simulink model "source"  (R2024b)
settings: Solver=ode15s  StartTime=0.0  StopTime=20  MaxStep=base.Ts  RelTol=1e-3  AbsTol=1e-4
values from neighbouring files (symbols this model uses):
  base = evalin("base", "base")    [base_wheel_state_space.m]    (also in build_base_nmpc_solver.m; configure_base_tracking_case.m; coupled_two_leg_qp_core.m; full_base_nmpc_state_signal.m)
  baseNmpc = evalin("base", "baseNmpc")    [base_nmpc_reference.m]    (also in build_base_nmpc_solver.m; configure_base_nmpc_simulink.m; configure_base_tracking_case.m; coupled_two_leg_qp_core.m)
  ctrl = evalin("base", "ctrl")    [coupled_two_leg_qp_core.m]    (also in full_base_nmpc_state_signal.m; set_initial_base_state.m; spatial_two_leg_qp_core.m; startup.m = struct())
  leg = evalin("base", "leg")    [base_wheel_state_space.m]    (also in build_base_nmpc_solver.m; coupled_two_leg_qp_core.m; full_base_nmpc_state_signal.m; full_base_wheel_state_space.m)
  m = fullBaseNmpc.model.m    [full_base_nmpc_ocp.m]
  N = baseNmpc.N    [base_nmpc_reference.m]    (also in full_base_nmpc_reference.m = config.N)
undefined symbols (not defined in the file or in its folder): X, Y, Z
libraries: sm_lib x30, nesl_utility x30
settings Model: Creator=Tan Dachao  LastModifiedBy=Tan Dachao
settings DataIOCC: LimitDataPoints=on  MaxDataPoints=20000  SaveOutput=off  DSMLogging=off  SaveTime=off
settings SimscapeCC: SimscapeLogType=all

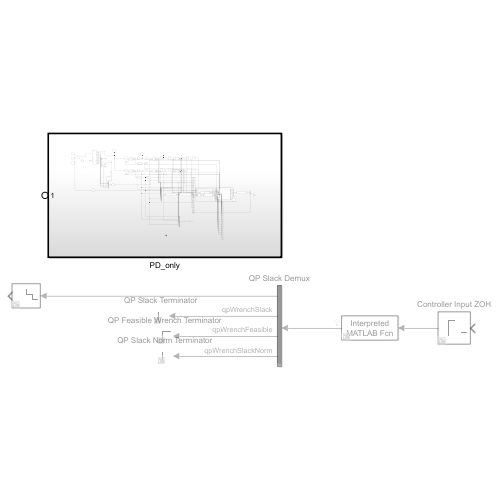
[thumbnail: Simulink's stored preview of the top-level diagram]
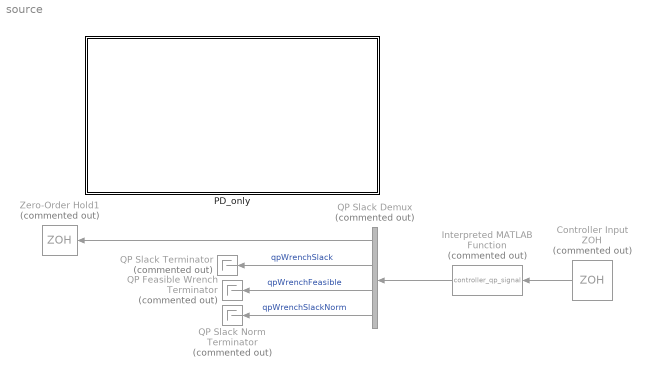
== system source ==
  Controller Input ZOH : ZeroOrderHold  Commented=on  SampleTime=base.Ts
  Interpreted MATLAB Function : MATLABFcn  Commented=on  MATLABFcn=controller_qp_signal  OutputDimensions=10  SampleTime=base.Ts
  PD_only : Subsystem  TreatAsAtomicUnit=on
      settings: MinAlgLoopOccurrences=on
  QP Feasible Wrench Terminator : Terminator  Commented=on
  QP Slack Demux : Demux  Commented=on  Outputs=[3 3 3 1]
  QP Slack Norm Terminator : Terminator  Commented=on
  QP Slack Terminator : Terminator  Commented=on
  Zero-Order Hold1 : ZeroOrderHold  Commented=on  SampleTime=base.Ts
  wires:
  Controller Input ZOH/1 -> Interpreted MATLAB Function/1
  Interpreted MATLAB Function/1 -> QP Slack Demux/1
  QP Slack Demux/1 -> Zero-Order Hold1/1
  QP Slack Demux/2 -> QP Slack Terminator/1  "qpWrenchSlack"
  QP Slack Demux/3 -> QP Feasible Wrench Terminator/1  "qpWrenchFeasible"
  QP Slack Demux/4 -> QP Slack Norm Terminator/1  "qpWrenchSlackNorm"

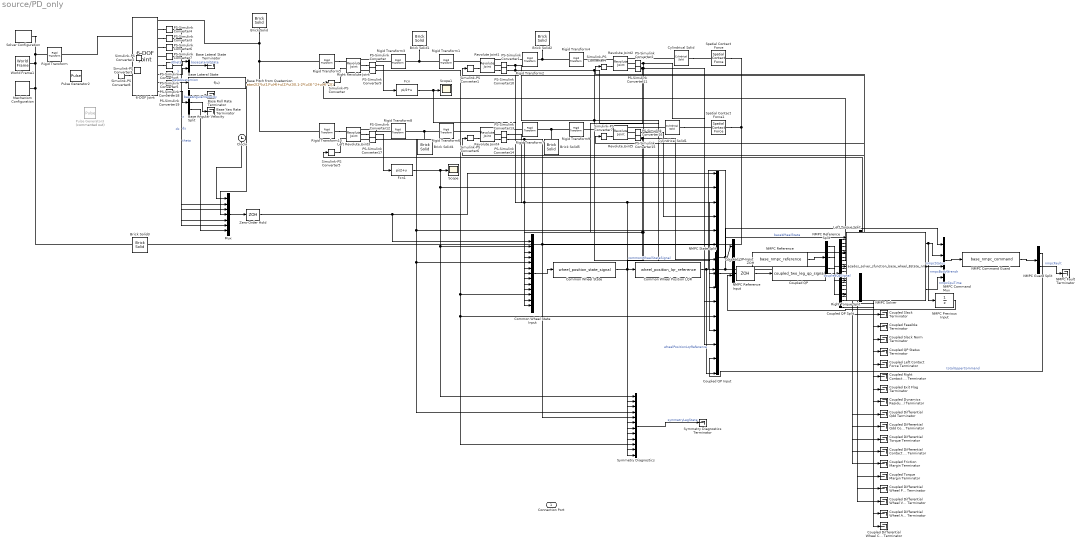
== system source/PD_only ==
  6-DOF Joint : sm_lib/Joints/6-DOF Joint  JointMode=Normal  CompositeWrenchDir=FollowerOnBase  CompositeWrenchFrame=BaseFrame  SenseConstraintForce=off  SenseConstraintTorque=off  SenseTotalForce=off  SenseTotalTorque=off  PxPositionTargetSpecify=on  PxPositionTargetPriority=High  PxPositionTargetValue=base.x0(1)  PxPositionTargetValueUnits=m  PxVelocityTargetSpecify=on  PxVelocityTargetPriority=High  PxVelocityTargetValue=base.x0(4)  PxVelocityTargetValueUnits=m/s  PxEquilibriumPosition=0  PxEquilibriumPositionUnits=m  PxSpringStiffness=0  PxSpringStiffnessUnits=N/m  PxDampingCoefficient=0  PxDampingCoefficientUnits=N/(m/s)  PxLowerLimitSpecify=off  PxLowerLimitBound=-1  PxLowerLimitBoundUnits=m  PxLowerLimitStiffness=1e6  PxLowerLimitStiffnessUnits=N/m  PxLowerLimitDamping=1e3  PxLowerLimitDampingUnits=N/(m/s)  PxLowerLimitTransitionRegionWidth=1e-4  PxLowerLimitTransitionRegionWidthUnits=m  PxUpperLimitSpecify=off  PxUpperLimitBound=1  PxUpperLimitBoundUnits=m  PxUpperLimitStiffness=1e6  PxUpperLimitStiffnessUnits=N/m  PxUpperLimitDamping=1e3  PxUpperLimitDampingUnits=N/(m/s)  PxUpperLimitTransitionRegionWidth=1e-4  PxUpperLimitTransitionRegionWidthUnits=m  PxTorqueActuationMode=InputTorque  PxMotionActuationMode=ComputedMotion  PxSensePosition=on  PxSenseVelocity=on  PxSenseAcceleration=off  PxSenseTorqueForce=off  PxSenseLowerLimitTorqueForce=off  PxSenseUpperLimitTorqueForce=off  PyPositionTargetSpecify=on  PyPositionTargetPriority=High  PyPositionTargetValue=base.x0(2)  PyPositionTargetValueUnits=m  PyVelocityTargetSpecify=on  PyVelocityTargetPriority=High  PyVelocityTargetValue=base.x0(5)  PyVelocityTargetValueUnits=m/s  PyEquilibriumPosition=0  PyEquilibriumPositionUnits=m  PySpringStiffness=0  PySpringStiffnessUnits=N/m  PyDampingCoefficient=0  PyDampingCoefficientUnits=N/(m/s)  PyLowerLimitSpecify=off  PyLowerLimitBound=-1  PyLowerLimitBoundUnits=m  PyLowerLimitStiffness=1e6  PyLowerLimitStiffnessUnits=N/m  PyLowerLimitDamping=1e3  PyLowerLimitDampingUnits=N/(m/s)  PyLowerLimitTransitionRegionWidth=1e-4  PyLowerLimitTransitionRegionWidthUnits=m  PyUpperLimitSpecify=off  PyUpperLimitBound=1  PyUpperLimitBoundUnits=m  PyUpperLimitStiffness=1e6  PyUpperLimitStiffnessUnits=N/m  PyUpperLimitDamping=1e3  PyUpperLimitDampingUnits=N/(m/s)  PyUpperLimitTransitionRegionWidth=1e-4  PyUpperLimitTransitionRegionWidthUnits=m  PyTorqueActuationMode=NoTorque  PyMotionActuationMode=ComputedMotion  PySensePosition=on  PySenseVelocity=on  PySenseAcceleration=off  PySenseTorqueForce=off  PySenseLowerLimitTorqueForce=off  PySenseUpperLimitTorqueForce=off  PzPositionTargetSpecify=on  PzPositionTargetPriority=High  PzPositionTargetValue=0  PzPositionTargetValueUnits=m  PzVelocityTargetSpecify=on  PzVelocityTargetPriority=High  PzVelocityTargetValue=0  PzVelocityTargetValueUnits=m/s  PzEquilibriumPosition=0  PzEquilibriumPositionUnits=m  PzSpringStiffness=0  PzSpringStiffnessUnits=N/m  PzDampingCoefficient=0  PzDampingCoefficientUnits=N/(m/s)  PzLowerLimitSpecify=off  PzLowerLimitBound=-1  PzLowerLimitBoundUnits=m  PzLowerLimitStiffness=1e6  PzLowerLimitStiffnessUnits=N/m  PzLowerLimitDamping=1e3  PzLowerLimitDampingUnits=N/(m/s)  PzLowerLimitTransitionRegionWidth=1e-4  PzLowerLimitTransitionRegionWidthUnits=m  PzUpperLimitSpecify=off  PzUpperLimitBound=1  PzUpperLimitBoundUnits=m  PzUpperLimitStiffness=1e6  PzUpperLimitStiffnessUnits=N/m  PzUpperLimitDamping=1e3  PzUpperLimitDampingUnits=N/(m/s)  PzUpperLimitTransitionRegionWidth=1e-4  PzUpperLimitTransitionRegionWidthUnits=m  PzTorqueActuationMode=NoTorque  PzMotionActuationMode=ComputedMotion  PzSensePosition=on  PzSenseVelocity=on  PzSenseAcceleration=off  PzSenseTorqueForce=off  PzSenseLowerLimitTorqueForce=off  PzSenseUpperLimitTorqueForce=off  SphPositionTargetSpecify=on  SphPositionTargetPriority=High  SphPositionTargetRotationMethod=Quaternion  SphPositionTargetFollAlignAxisA=+X  SphPositionTargetBaseAlignAxisA=+Y  SphPositionTargetFollAlignAxisB=+Y  SphPositionTargetBaseAlignAxisB=+Z  SphPositionTargetRotationStandardAxis=+Z  SphPositionTargetRotationAngle=0  SphPositionTargetRotationAngleUnits=deg  SphPositionTargetRotationArbitraryAxis=[0 0 1]  SphPositionTargetRotationSequenceAxes=FollowerAxes  SphPositionTargetRotationSequence=XYX  SphPositionTargetRotationSequenceAngles=[0 0 0]  SphPositionTargetRotationSequenceAnglesUnits=deg  SphPositionTargetRotationMatrix=[1 0 0;0 1 0;0 0 1]  SphPositionTargetQuaternion=[cos(base.x0(3)/2) 0 0 sin(base.x0(3)/2)]  SphVelocityTargetSpecify=on  SphVelocityTargetPriority=High  SphVelocityTargetValue=[0 0 base.x0(6)]  SphVelocityTargetValueUnits=deg/s  SphVelocityTargetInFollowerFrame=off  SphEqPosRotationMethod=None  SphEqPosFollAlignAxisA=+X  SphEqPosBaseAlignAxisA=+Y  SphEqPosFollAlignAxisB=+Y  SphEqPosBaseAlignAxisB=+Z  SphEqPosRotationStandardAxis=+Z  SphEqPosRotationAngle=0  SphEqPosRotationAngleUnits=deg  SphEqPosRotationArbitraryAxis=[0 0 1]  SphEqPosRotationSequenceAxes=FollowerAxes  SphEqPosRotationSequence=XYX  SphEqPosRotationSequenceAngles=[0 0 0]  SphEqPosRotationSequenceAnglesUnits=deg  SphEqPosRotationMatrix=[1 0 0;0 1 0;0 0 1]  SphEqPosQuaternion=[1 0 0 0]  SphSpringStiffness=0  SphSpringStiffnessUnits=N*m/deg  SphDampingCoefficient=0  SphDampingCoefficientUnits=N*m/(deg/s)  SphLowerLimitSpecify=off  SphLowerLimitBound=15  SphLowerLimitBoundUnits=deg  SphLowerLimitStiffness=1e4  SphLowerLimitStiffnessUnits=N*m/deg  SphLowerLimitDamping=10  SphLowerLimitDampingUnits=N*m/(deg/s)  SphLowerLimitTransitionRegionWidth=0.1  SphLowerLimitTransitionRegionWidthUnits=deg  SphUpperLimitSpecify=off  SphUpperLimitBound=45  SphUpperLimitBoundUnits=deg  SphUpperLimitStiffness=1e4  SphUpperLimitStiffnessUnits=N*m/deg  SphUpperLimitDamping=10  SphUpperLimitDampingUnits=N*m/(deg/s)  SphUpperLimitTransitionRegionWidth=0.1  SphUpperLimitTransitionRegionWidthUnits=deg  SphTorqueActuationMode=NoTorque  SphActuateTorqueX=off  SphActuateTorqueY=off  SphActuateTorqueZ=off  SphActuateTorque=off  SphActuationFrame=BaseFrame  SphSensePosition=on  SphSenseVelocityX=off  SphSenseVelocityY=off  SphSenseVelocityZ=off  SphSenseVelocity=on  SphSenseAccelerationX=off  SphSenseAccelerationY=off  SphSenseAccelerationZ=off  SphSenseAcceleration=off  SphSenseLowerLimitTorqueMag=off  SphSenseUpperLimitTorqueMag=off  SphSensingFrame=BaseFrame
  Base Angular Velocity Split : Demux  Outputs=3
  Base Lateral State : Mux  Inputs=2
  Base Lateral State Terminator : Terminator
  Base Pitch from Quaternion : Fcn  Expr=atan2(2*(u(1)*u(4)+u(2)*u(3)),1-2*(u(3)^2+u(4)^2))
  Base Roll Rate Terminator : Terminator
  Base Yaw Rate Terminator : Terminator
  Brick Solid : sm_lib/Body Elements/Brick Solid  BrickDimensions=[0.45 0.32 0.45]  BrickDimensionsUnits=m  ExportEntireGeometry=off  InertiaType=CalculateFromGeometry  BasedOnType=Mass  Density=1000  DensityUnits=kg/m^3  Mass=3  MassUnits=kg  CenterOfMass=[0 0 0]  CenterOfMassUnits=m  MomentsOfInertia=[1 1 1]  MomentsOfInertiaUnits=kg*m^2  ProductsOfInertia=[0 0 0]  ProductsOfInertiaUnits=kg*m^2  GraphicType=FromGeometry  MarkerShape=Sphere  MarkerSize=10  GraphicVisPropType=SimpleVisualProperties  GraphicDiffuseColor=[0.5 0.5 0.5]  GraphicOpacity=1  GraphicSpecularColor=[0.5 0.5 0.5 1.0]  GraphicAmbientColor=[0.15 0.15 0.15 1.0]  GraphicEmissiveColor=[0.0 0.0 0.0 1.0]  GraphicShininess=75  DoExposeReferenceFrame=on  SerializedFrames=<Frames/>
  Brick Solid1 : sm_lib/Body Elements/Brick Solid  BrickDimensions=[0.35 0.04 .04]  BrickDimensionsUnits=m  ExportEntireGeometry=off  InertiaType=CalculateFromGeometry  BasedOnType=Mass  Density=1000  DensityUnits=kg/m^3  Mass=1.20  MassUnits=kg  CenterOfMass=[0 0 0]  CenterOfMassUnits=m  MomentsOfInertia=[1 1 1]  MomentsOfInertiaUnits=kg*m^2  ProductsOfInertia=[0 0 0]  ProductsOfInertiaUnits=kg*m^2  GraphicType=FromGeometry  MarkerShape=Sphere  MarkerSize=10  GraphicVisPropType=SimpleVisualProperties  GraphicDiffuseColor=[0.5 0.5 0.5]  GraphicOpacity=1  GraphicSpecularColor=[0.5 0.5 0.5 1.0]  GraphicAmbientColor=[0.15 0.15 0.15 1.0]  GraphicEmissiveColor=[0.0 0.0 0.0 1.0]  GraphicShininess=75  DoExposeReferenceFrame=on  SerializedFrames=<Frames/>
  Brick Solid2 : sm_lib/Body Elements/Brick Solid  BrickDimensions=[0.35 0.04 .04]  BrickDimensionsUnits=m  ExportEntireGeometry=off  InertiaType=CalculateFromGeometry  BasedOnType=Mass  Density=1000  DensityUnits=kg/m^3  Mass=0.8  MassUnits=kg  CenterOfMass=[0 0 0]  CenterOfMassUnits=m  MomentsOfInertia=[1 1 1]  MomentsOfInertiaUnits=kg*m^2  ProductsOfInertia=[0 0 0]  ProductsOfInertiaUnits=kg*m^2  GraphicType=FromGeometry  MarkerShape=Sphere  MarkerSize=10  GraphicVisPropType=SimpleVisualProperties  GraphicDiffuseColor=[0.5 0.5 0.5]  GraphicOpacity=1  GraphicSpecularColor=[0.5 0.5 0.5 1.0]  GraphicAmbientColor=[0.15 0.15 0.15 1.0]  GraphicEmissiveColor=[0.0 0.0 0.0 1.0]  GraphicShininess=75  DoExposeReferenceFrame=on  SerializedFrames=<Frames/>
  Brick Solid3 : sm_lib/Body Elements/Brick Solid  BrickDimensions=[15 .05 3]  BrickDimensionsUnits=m  ExportEntireGeometry=on  InertiaType=CalculateFromGeometry  BasedOnType=Mass  Density=1000  DensityUnits=kg/m^3  Mass=1  MassUnits=kg  CenterOfMass=[0 0 0]  CenterOfMassUnits=m  MomentsOfInertia=[1 1 1]  MomentsOfInertiaUnits=kg*m^2  ProductsOfInertia=[0 0 0]  ProductsOfInertiaUnits=kg*m^2  GraphicType=FromGeometry  MarkerShape=Sphere  MarkerSize=10  GraphicVisPropType=SimpleVisualProperties  GraphicDiffuseColor=[1 1 0.06667]  GraphicOpacity=1  GraphicSpecularColor=[0.5 0.5 0.5 1.0]  GraphicAmbientColor=[0.15 0.15 0.15 1.0]  GraphicEmissiveColor=[0.0 0.0 0.0 1.0]  GraphicShininess=75  DoExposeReferenceFrame=on  SerializedFrames=<Frames/>
  Brick Solid4 : sm_lib/Body Elements/Brick Solid  BrickDimensions=[0.35 0.04 .04]  BrickDimensionsUnits=m  ExportEntireGeometry=off  InertiaType=CalculateFromGeometry  BasedOnType=Mass  Density=1000  DensityUnits=kg/m^3  Mass=1.20  MassUnits=kg  CenterOfMass=[0 0 0]  CenterOfMassUnits=m  MomentsOfInertia=[1 1 1]  MomentsOfInertiaUnits=kg*m^2  ProductsOfInertia=[0 0 0]  ProductsOfInertiaUnits=kg*m^2  GraphicType=FromGeometry  MarkerShape=Sphere  MarkerSize=10  GraphicVisPropType=SimpleVisualProperties  GraphicDiffuseColor=[0.5 0.5 0.5]  GraphicOpacity=1  GraphicSpecularColor=[0.5 0.5 0.5 1.0]  GraphicAmbientColor=[0.15 0.15 0.15 1.0]  GraphicEmissiveColor=[0.0 0.0 0.0 1.0]  GraphicShininess=75  DoExposeReferenceFrame=on  SerializedFrames=<Frames/>
  Brick Solid5 : sm_lib/Body Elements/Brick Solid  BrickDimensions=[0.35 0.04 .04]  BrickDimensionsUnits=m  ExportEntireGeometry=off  InertiaType=CalculateFromGeometry  BasedOnType=Mass  Density=1000  DensityUnits=kg/m^3  Mass=0.8  MassUnits=kg  CenterOfMass=[0 0 0]  CenterOfMassUnits=m  MomentsOfInertia=[1 1 1]  MomentsOfInertiaUnits=kg*m^2  ProductsOfInertia=[0 0 0]  ProductsOfInertiaUnits=kg*m^2  GraphicType=FromGeometry  MarkerShape=Sphere  MarkerSize=10  GraphicVisPropType=SimpleVisualProperties  GraphicDiffuseColor=[0.5 0.5 0.5]  GraphicOpacity=1  GraphicSpecularColor=[0.5 0.5 0.5 1.0]  GraphicAmbientColor=[0.15 0.15 0.15 1.0]  GraphicEmissiveColor=[0.0 0.0 0.0 1.0]  GraphicShininess=75  DoExposeReferenceFrame=on  SerializedFrames=<Frames/>
  Clock : Clock
  Common Wheel Position LQR : MATLABFcn  MATLABFcn=wheel_position_lqr_reference  OutputDimensions=4  SampleTime=base.Ts
  Common Wheel State : MATLABFcn  MATLABFcn=wheel_position_state_signal  OutputDimensions=10  SampleTime=base.Ts
  Common Wheel State Input : Mux  Inputs=13
  Coupled Differential Contact Force Terminator : Terminator
  Coupled Differential Qdd Command Terminator : Terminator
  Coupled Differential Qdd Terminator : Terminator
  Coupled Differential Torque Terminator : Terminator
  Coupled Differential Wheel Acceleration Terminator : Terminator
  Coupled Differential Wheel Command Terminator : Terminator
  Coupled Differential Wheel Position Terminator : Terminator
  Coupled Differential Wheel Velocity Terminator : Terminator
  Coupled Dynamics Residual Terminator : Terminator
  Coupled Exit Flag Terminator : Terminator
  Coupled Feasible Terminator : Terminator
  Coupled Friction Margin Terminator : Terminator
  Coupled Left Contact Force Terminator : Terminator
  Coupled QP : MATLABFcn  MATLABFcn=coupled_two_leg_qp_signal  OutputDimensions=43  SampleTime=base.Ts
  Coupled QP Input : Mux  Inputs=15
  Coupled QP Input ZOH : ZeroOrderHold  SampleTime=base.Ts
  Coupled QP Split : Demux  Outputs=[3 3 3 3 1 1 2 2 1 1 3 3 3 2 2 6 1 1 1 1]
  Coupled QP Status Terminator : Terminator
  Coupled Right Contact Force Terminator : Terminator
  Coupled Slack Norm Terminator : Terminator
  Coupled Slack Terminator : Terminator
  Coupled Torque Margin Terminator : Terminator
  Cylindrical Solid : sm_lib/Body Elements/Cylindrical Solid  CylinderRadius=0.08  CylinderRadiusUnits=m  CylinderLength=0.1  CylinderLengthUnits=m  ExportEntireGeometry=on  InertiaType=CalculateFromGeometry  BasedOnType=Mass  Density=1000  DensityUnits=kg/m^3  Mass=0.35  MassUnits=kg  CenterOfMass=[0 0 0]  CenterOfMassUnits=m  MomentsOfInertia=[1 1 1]  MomentsOfInertiaUnits=kg*m^2  ProductsOfInertia=[0 0 0]  ProductsOfInertiaUnits=kg*m^2  GraphicType=FromGeometry  MarkerShape=Sphere  MarkerSize=10  GraphicVisPropType=AdvancedVisualProperties  GraphicDiffuseColor=[0 1 0]  GraphicOpacity=1  GraphicSpecularColor=[0.5 0.5 0.5 0.3]  GraphicAmbientColor=[0.15 0.15 0.15 0.3]  GraphicEmissiveColor=[0.0 0.0 0.0 0.3]  GraphicShininess=1  DoExposeReferenceFrame=on  SerializedFrames=<Frames/>
  Cylindrical Solid1 : sm_lib/Body Elements/Cylindrical Solid  CylinderRadius=0.08  CylinderRadiusUnits=m  CylinderLength=0.1  CylinderLengthUnits=m  ExportEntireGeometry=on  InertiaType=CalculateFromGeometry  BasedOnType=Mass  Density=1000  DensityUnits=kg/m^3  Mass=0.35  MassUnits=kg  CenterOfMass=[0 0 0]  CenterOfMassUnits=m  MomentsOfInertia=[1 1 1]  MomentsOfInertiaUnits=kg*m^2  ProductsOfInertia=[0 0 0]  ProductsOfInertiaUnits=kg*m^2  GraphicType=FromGeometry  MarkerShape=Sphere  MarkerSize=10  GraphicVisPropType=AdvancedVisualProperties  GraphicDiffuseColor=[0 1 0]  GraphicOpacity=1  GraphicSpecularColor=[0.5 0.5 0.5 0.3]  GraphicAmbientColor=[0.15 0.15 0.15 0.3]  GraphicEmissiveColor=[0.0 0.0 0.0 0.3]  GraphicShininess=1  DoExposeReferenceFrame=on  SerializedFrames=<Frames/>
  Fcn : Fcn  Expr=pi/2+u
  Fcn1 : Fcn  Expr=pi/2+u
  Left Revolute Joint3 : sm_lib/Joints/Revolute Joint  JointMode=Normal  CompositeWrenchDir=FollowerOnBase  CompositeWrenchFrame=BaseFrame  SenseConstraintForce=off  SenseConstraintTorque=off  SenseTotalForce=off  SenseTotalTorque=off  PositionTargetSpecify=on  PositionTargetPriority=High  PositionTargetValue=leg.q0(1)-pi/2  PositionTargetValueUnits=rad  VelocityTargetSpecify=on  VelocityTargetPriority=High  VelocityTargetValue=0  VelocityTargetValueUnits=rad/s  EquilibriumPosition=0  EquilibriumPositionUnits=deg  SpringStiffness=0  SpringStiffnessUnits=N*m/deg  DampingCoefficient=ctrl.commonModeJointDamping(1)  DampingCoefficientUnits=N*m/(rad/s)  LowerLimitSpecify=off  LowerLimitBound=-90  LowerLimitBoundUnits=deg  LowerLimitStiffness=1e4  LowerLimitStiffnessUnits=N*m/deg  LowerLimitDamping=10  LowerLimitDampingUnits=N*m/(deg/s)  LowerLimitTransitionRegionWidth=0.1  LowerLimitTransitionRegionWidthUnits=deg  UpperLimitSpecify=off  UpperLimitBound=90  UpperLimitBoundUnits=deg  UpperLimitStiffness=1e4  UpperLimitStiffnessUnits=N*m/deg  UpperLimitDamping=10  UpperLimitDampingUnits=N*m/(deg/s)  UpperLimitTransitionRegionWidth=0.1  UpperLimitTransitionRegionWidthUnits=deg  TorqueActuationMode=InputTorque  MotionActuationMode=ComputedMotion  SensePosition=on  SenseVelocity=on  SenseAcceleration=off  SenseTorqueForce=off  SenseLowerLimitTorqueForce=off  SenseUpperLimitTorqueForce=off
  Left Torque Split : Demux  Outputs=3
  Mechanism Configuration : sm_lib/Utilities/Mechanism Configuration  UniformGravity=Constant  GravityVector=[0 -9.81 0]  GravityVectorUnits=m/s^2  LinearizationDelta=0.001  JointModeTransitionNonlinearIterations=2
  Mux : Mux  Inputs=7
  NMPC Command Guard : MATLABFcn  MATLABFcn=base_nmpc_command  OutputDimensions=4  SampleTime=baseNmpc.Ts
  NMPC Command Mux : Mux
  NMPC Fault Terminator : Terminator
  NMPC Guard Split : Demux  Outputs=[3 1]
  NMPC Previous Input : UnitDelay  InitialCondition=baseNmpc.model.uEq  SampleTime=baseNmpc.Ts  HasFrameUpgradeWarning=on
  NMPC Reference : MATLABFcn  MATLABFcn=base_nmpc_reference  OutputDimensions=428  SampleTime=baseNmpc.Ts
  NMPC Reference Input : Mux  Inputs=3
  NMPC Reference Split : Demux  Outputs=[14 406 8]
  NMPC Solver : S-Function  FunctionName=acados_solver_sfunction_base_wheel_8state_nmpc  SFunctionDeploymentMode=off  EnableBusSupport=off
      mask Display:
      | port_label('input', 1, 'lbx_0 [8]')
      | port_label('input', 2, 'ubx_0 [8]')
      | port_label('input', 3, 'y_ref_0 [14]')
      | port_label('input', 4, 'y_ref [406]')
      | port_label('input', 5, 'y_ref_e [8]')
      | port_label('output', 1, 'u0 [3]')
      | port_label('output', 2, 'solver_status')
      | port_label('output', 3, 'CPU_time')
      | disp('base_wheel_8state_nmpc acados OCP')
  NMPC State Split : Demux  Outputs=[1 8 1]
  PS-Simulink Converter{,1..19} (20 alike) : nesl_utility/PS-Simulink Converter  PhysicalDomain=network_engine_domain  SubClassName=ps_output  LeftPortType=input  RightPortType=output  PseudoPeriodic=off  Frequencies=[]  VectorFormat=inherit  Unit=inherit  AffineConversion=off
  Pulse Generator2 : DiscretePulseGenerator  PulseType=Time based  Amplitude=15  Period=10  PulseWidth=5  PhaseDelay=2.5
  Pulse Generator3 : DiscretePulseGenerator  Commented=on  PulseType=Time based  Amplitude=0  Period=10  PulseWidth=80  PhaseDelay=5
  Revolute Joint1 : sm_lib/Joints/Revolute Joint  JointMode=Normal  CompositeWrenchDir=FollowerOnBase  CompositeWrenchFrame=BaseFrame  SenseConstraintForce=off  SenseConstraintTorque=off  SenseTotalForce=off  SenseTotalTorque=off  PositionTargetSpecify=on  PositionTargetPriority=High  PositionTargetValue=leg.q0(2)  PositionTargetValueUnits=rad  VelocityTargetSpecify=on  VelocityTargetPriority=High  VelocityTargetValue=0  VelocityTargetValueUnits=rad/s  EquilibriumPosition=0  EquilibriumPositionUnits=deg  SpringStiffness=0  SpringStiffnessUnits=N*m/deg  DampingCoefficient=ctrl.commonModeJointDamping(2)  DampingCoefficientUnits=N*m/(rad/s)  LowerLimitSpecify=off  LowerLimitBound=-90  LowerLimitBoundUnits=deg  LowerLimitStiffness=1e4  LowerLimitStiffnessUnits=N*m/deg  LowerLimitDamping=10  LowerLimitDampingUnits=N*m/(deg/s)  LowerLimitTransitionRegionWidth=0.1  LowerLimitTransitionRegionWidthUnits=deg  UpperLimitSpecify=off  UpperLimitBound=90  UpperLimitBoundUnits=deg  UpperLimitStiffness=1e4  UpperLimitStiffnessUnits=N*m/deg  UpperLimitDamping=10  UpperLimitDampingUnits=N*m/(deg/s)  UpperLimitTransitionRegionWidth=0.1  UpperLimitTransitionRegionWidthUnits=deg  TorqueActuationMode=InputTorque  MotionActuationMode=ComputedMotion  SensePosition=on  SenseVelocity=on  SenseAcceleration=off  SenseTorqueForce=off  SenseLowerLimitTorqueForce=off  SenseUpperLimitTorqueForce=off
  Revolute Joint2 : sm_lib/Joints/Revolute Joint  JointMode=Normal  CompositeWrenchDir=FollowerOnBase  CompositeWrenchFrame=BaseFrame  SenseConstraintForce=off  SenseConstraintTorque=off  SenseTotalForce=off  SenseTotalTorque=off  PositionTargetSpecify=on  PositionTargetPriority=High  PositionTargetValue=leg.q0(3)  PositionTargetValueUnits=rad  VelocityTargetSpecify=on  VelocityTargetPriority=High  VelocityTargetValue=0  VelocityTargetValueUnits=rad/s  EquilibriumPosition=0  EquilibriumPositionUnits=deg  SpringStiffness=0  SpringStiffnessUnits=N*m/deg  DampingCoefficient=ctrl.commonModeJointDamping(3)  DampingCoefficientUnits=N*m/(rad/s)  LowerLimitSpecify=off  LowerLimitBound=-90  LowerLimitBoundUnits=deg  LowerLimitStiffness=1e4  LowerLimitStiffnessUnits=N*m/deg  LowerLimitDamping=10  LowerLimitDampingUnits=N*m/(deg/s)  LowerLimitTransitionRegionWidth=0.1  LowerLimitTransitionRegionWidthUnits=deg  UpperLimitSpecify=off  UpperLimitBound=90  UpperLimitBoundUnits=deg  UpperLimitStiffness=1e4  UpperLimitStiffnessUnits=N*m/deg  UpperLimitDamping=10  UpperLimitDampingUnits=N*m/(deg/s)  UpperLimitTransitionRegionWidth=0.1  UpperLimitTransitionRegionWidthUnits=deg  TorqueActuationMode=InputTorque  MotionActuationMode=ComputedMotion  SensePosition=on  SenseVelocity=on  SenseAcceleration=off  SenseTorqueForce=off  SenseLowerLimitTorqueForce=off  SenseUpperLimitTorqueForce=off
  Revolute Joint4 : sm_lib/Joints/Revolute Joint  JointMode=Normal  CompositeWrenchDir=FollowerOnBase  CompositeWrenchFrame=BaseFrame  SenseConstraintForce=off  SenseConstraintTorque=off  SenseTotalForce=off  SenseTotalTorque=off  PositionTargetSpecify=on  PositionTargetPriority=High  PositionTargetValue=leg.q0(2)  PositionTargetValueUnits=rad  VelocityTargetSpecify=on  VelocityTargetPriority=High  VelocityTargetValue=0  VelocityTargetValueUnits=rad/s  EquilibriumPosition=0  EquilibriumPositionUnits=deg  SpringStiffness=0  SpringStiffnessUnits=N*m/deg  DampingCoefficient=ctrl.commonModeJointDamping(2)  DampingCoefficientUnits=N*m/(rad/s)  LowerLimitSpecify=off  LowerLimitBound=-90  LowerLimitBoundUnits=deg  LowerLimitStiffness=1e4  LowerLimitStiffnessUnits=N*m/deg  LowerLimitDamping=10  LowerLimitDampingUnits=N*m/(deg/s)  LowerLimitTransitionRegionWidth=0.1  LowerLimitTransitionRegionWidthUnits=deg  UpperLimitSpecify=off  UpperLimitBound=90  UpperLimitBoundUnits=deg  UpperLimitStiffness=1e4  UpperLimitStiffnessUnits=N*m/deg  UpperLimitDamping=10  UpperLimitDampingUnits=N*m/(deg/s)  UpperLimitTransitionRegionWidth=0.1  UpperLimitTransitionRegionWidthUnits=deg  TorqueActuationMode=InputTorque  MotionActuationMode=ComputedMotion  SensePosition=on  SenseVelocity=on  SenseAcceleration=off  SenseTorqueForce=off  SenseLowerLimitTorqueForce=off  SenseUpperLimitTorqueForce=off
  Revolute Joint5 : sm_lib/Joints/Revolute Joint  JointMode=Normal  CompositeWrenchDir=FollowerOnBase  CompositeWrenchFrame=BaseFrame  SenseConstraintForce=off  SenseConstraintTorque=off  SenseTotalForce=off  SenseTotalTorque=off  PositionTargetSpecify=on  PositionTargetPriority=High  PositionTargetValue=leg.q0(3)  PositionTargetValueUnits=rad  VelocityTargetSpecify=on  VelocityTargetPriority=High  VelocityTargetValue=0  VelocityTargetValueUnits=rad/s  EquilibriumPosition=0  EquilibriumPositionUnits=deg  SpringStiffness=0  SpringStiffnessUnits=N*m/deg  DampingCoefficient=ctrl.commonModeJointDamping(3)  DampingCoefficientUnits=N*m/(rad/s)  LowerLimitSpecify=off  LowerLimitBound=-90  LowerLimitBoundUnits=deg  LowerLimitStiffness=1e4  LowerLimitStiffnessUnits=N*m/deg  LowerLimitDamping=10  LowerLimitDampingUnits=N*m/(deg/s)  LowerLimitTransitionRegionWidth=0.1  LowerLimitTransitionRegionWidthUnits=deg  UpperLimitSpecify=off  UpperLimitBound=90  UpperLimitBoundUnits=deg  UpperLimitStiffness=1e4  UpperLimitStiffnessUnits=N*m/deg  UpperLimitDamping=10  UpperLimitDampingUnits=N*m/(deg/s)  UpperLimitTransitionRegionWidth=0.1  UpperLimitTransitionRegionWidthUnits=deg  TorqueActuationMode=InputTorque  MotionActuationMode=ComputedMotion  SensePosition=on  SenseVelocity=on  SenseAcceleration=off  SenseTorqueForce=off  SenseLowerLimitTorqueForce=off  SenseUpperLimitTorqueForce=off
  Right Revolute Joint : sm_lib/Joints/Revolute Joint  JointMode=Normal  CompositeWrenchDir=FollowerOnBase  CompositeWrenchFrame=BaseFrame  SenseConstraintForce=off  SenseConstraintTorque=off  SenseTotalForce=off  SenseTotalTorque=off  PositionTargetSpecify=on  PositionTargetPriority=High  PositionTargetValue=leg.q0(1)-pi/2  PositionTargetValueUnits=rad  VelocityTargetSpecify=on  VelocityTargetPriority=High  VelocityTargetValue=0  VelocityTargetValueUnits=rad/s  EquilibriumPosition=0  EquilibriumPositionUnits=deg  SpringStiffness=0  SpringStiffnessUnits=N*m/deg  DampingCoefficient=ctrl.commonModeJointDamping(1)  DampingCoefficientUnits=N*m/(rad/s)  LowerLimitSpecify=off  LowerLimitBound=-90  LowerLimitBoundUnits=deg  LowerLimitStiffness=1e4  LowerLimitStiffnessUnits=N*m/deg  LowerLimitDamping=10  LowerLimitDampingUnits=N*m/(deg/s)  LowerLimitTransitionRegionWidth=0.1  LowerLimitTransitionRegionWidthUnits=deg  UpperLimitSpecify=off  UpperLimitBound=90  UpperLimitBoundUnits=deg  UpperLimitStiffness=1e4  UpperLimitStiffnessUnits=N*m/deg  UpperLimitDamping=10  UpperLimitDampingUnits=N*m/(deg/s)  UpperLimitTransitionRegionWidth=0.1  UpperLimitTransitionRegionWidthUnits=deg  TorqueActuationMode=InputTorque  MotionActuationMode=ComputedMotion  SensePosition=on  SenseVelocity=on  SenseAcceleration=off  SenseTorqueForce=off  SenseLowerLimitTorqueForce=off  SenseUpperLimitTorqueForce=off
  Right Torque Split : Demux  Outputs=3
  Rigid Transform : sm_lib/Frames and Transforms/Rigid Transform  RotationMethod=None  FollAlignAxisA=+X  BaseAlignAxisA=+Y  FollAlignAxisB=+Y  BaseAlignAxisB=+Z  RotationStandardAxis=+Z  RotationAngle=0  RotationAngleUnits=deg  RotationArbitraryAxis=[0 0 1]  RotationSequenceAxes=FollowerAxes  RotationSequence=XYX  RotationSequenceAngles=[0 0 0]  RotationSequenceAnglesUnits=deg  RotationMatrix=[1 0 0;0 1 0;0 0 1]  Quaternion=[1 0 0 0]  TranslationMethod=StandardAxis  TranslationCartesianOffset=[0 0 0]  TranslationCartesianOffsetUnits=m  TranslationStandardAxis=+Y  TranslationStandardOffset=base.simscapeWorldYOffset - ctrl.commonModeContactPreload  TranslationStandardOffsetUnits=m  TranslationROffset=0  TranslationROffsetUnits=m  TranslationThetaOffset=0  TranslationThetaOffsetUnits=deg  TranslationZOffset=0  TranslationZOffsetUnits=m
  Rigid Transform{1..4,6..9} (8 alike) : sm_lib/Frames and Transforms/Rigid Transform  RotationMethod=None  FollAlignAxisA=+X  BaseAlignAxisA=+Y  FollAlignAxisB=+Y  BaseAlignAxisB=+Z  RotationStandardAxis=+Z  RotationAngle=0  RotationAngleUnits=deg  RotationArbitraryAxis=[0 0 1]  RotationSequenceAxes=FollowerAxes  RotationSequence=XYX  RotationSequenceAngles=[0 0 0]  RotationSequenceAnglesUnits=deg  RotationMatrix=[1 0 0;0 1 0;0 0 1]  Quaternion=[1 0 0 0]  TranslationMethod=StandardAxis  TranslationCartesianOffset=[0 0 0]  TranslationCartesianOffsetUnits=m  TranslationStandardAxis=+X  TranslationStandardOffset=.175  TranslationStandardOffsetUnits=m  TranslationROffset=0  TranslationROffsetUnits=m  TranslationThetaOffset=0  TranslationThetaOffsetUnits=deg  TranslationZOffset=0  TranslationZOffsetUnits=m
  Rigid Transform10 : sm_lib/Frames and Transforms/Rigid Transform  RotationMethod=None  FollAlignAxisA=+X  BaseAlignAxisA=+Y  FollAlignAxisB=+Y  BaseAlignAxisB=+Z  RotationStandardAxis=+Z  RotationAngle=0  RotationAngleUnits=deg  RotationArbitraryAxis=[0 0 1]  RotationSequenceAxes=FollowerAxes  RotationSequence=XYX  RotationSequenceAngles=[0 0 0]  RotationSequenceAnglesUnits=deg  RotationMatrix=[1 0 0;0 1 0;0 0 1]  Quaternion=[1 0 0 0]  TranslationMethod=StandardAxis  TranslationCartesianOffset=[0 0 0]  TranslationCartesianOffsetUnits=m  TranslationStandardAxis=+Z  TranslationStandardOffset=-.2  TranslationStandardOffsetUnits=m  TranslationROffset=0  TranslationROffsetUnits=m  TranslationThetaOffset=0  TranslationThetaOffsetUnits=deg  TranslationZOffset=0  TranslationZOffsetUnits=m
  Rigid Transform5 : sm_lib/Frames and Transforms/Rigid Transform  RotationMethod=None  FollAlignAxisA=+X  BaseAlignAxisA=+Y  FollAlignAxisB=+Y  BaseAlignAxisB=+Z  RotationStandardAxis=+Z  RotationAngle=0  RotationAngleUnits=deg  RotationArbitraryAxis=[0 0 1]  RotationSequenceAxes=FollowerAxes  RotationSequence=XYX  RotationSequenceAngles=[0 0 0]  RotationSequenceAnglesUnits=deg  RotationMatrix=[1 0 0;0 1 0;0 0 1]  Quaternion=[1 0 0 0]  TranslationMethod=StandardAxis  TranslationCartesianOffset=[0 0 0]  TranslationCartesianOffsetUnits=m  TranslationStandardAxis=+Z  TranslationStandardOffset=.2  TranslationStandardOffsetUnits=m  TranslationROffset=0  TranslationROffsetUnits=m  TranslationThetaOffset=0  TranslationThetaOffsetUnits=deg  TranslationZOffset=0  TranslationZOffsetUnits=m
  Scope : Scope
  Scope1 : Scope
  Simulink-PS Converter{,1..8} (9 alike) : nesl_utility/Simulink-PS Converter  PhysicalDomain=network_engine_domain  SubClassName=ps_input  LeftPortType=input  RightPortType=output  PseudoPeriodic=off  Frequencies=[]  NoiseDistribution=none  NoiseParameters=[]  Unit=1  AffineConversion=off  FilteringAndDerivatives=provide  SimscapeFilterOrder=1  InputFilterTimeConstant=0.001  UdotUserProvided=0
  Solver Configuration : nesl_utility/Solver Configuration  PhysicalDomain=network_engine_domain  SubClassName=solver  LeftPortType=input  RightPortType=generic  Tones=[]  Harmonics=[]  SimulateNoise=off  Profile=off  UseLocalSampling=off  EnableSwitchedLinearOptims=on  FrequencyDomain=off  UseCCode=off  RelTol=0.001  AbsTol=0.001  MinStep=1e-09  ToWorkspace=off  RevertToSquareIcSolve=off  NumHomotopyIterations=100  PhasorMode=off  PhasorModeNumHarmonics=1  ConsistencySolver=NEWTON_XTOL_AFTER_FTOL  IndexReductionMethod=DerivativeReplacement  DoDC=off  ResidualTolerance=1e-09  ConsistencyTolSource=GLOBAL  ConsistencyAbsTol=0.001  ConsistencyRelTol=0.001  ConsistencyTolFactor=0.001  UseLocalSolver=off  LocalSolverChoice=NE_BACKWARD_EULER_ADVANCER  ResolveIndetEquations=on  FunctionEvalNumThread=1  LocalSolverSampleTime=0.001  DoFixedCost=off  MaxNonlinIter=3  MaxModeIter=2  ComputeImpulses=off  ImpulseIterations=2  LinearAlgebra=auto  LinearAlgebraNumThread=0  EquationFormulation=NE_TIME_EF  DelaysMemoryBudget=1024  AutomaticFiltering=on  FilteringTimeConstant=0.001  PartitionStorageMethod=AS_NEEDED  PartitionMemoryBudget=1024  PartitionMethod=ROBUST  MultibodyUseLocalSolver=off  MultibodyLocalSolverChoice=ODE1  MultibodyLocalSolverSampleTime=0.001
  Spatial Contact Force : sm_lib/Forces and Torques/Spatial Contact Force  NormalForceType=SmoothSpringDamper  NormalStiffness=ctrl.commonModeContactStiffness/2  NormalStiffnessUnits=N/m  NormalDamping=ctrl.commonModeContactDamping/2  NormalDampingUnits=N/(m/s)  NormalTransitionRegionWidth=1e-3  NormalTransitionRegionWidthUnits=m  FrictionType=SmoothStickSlip  CoefficientOfStaticFriction=0.5  CoefficientOfDynamicFriction=0.3  FrictionalCriticalVelocity=0.02  FrictionalCriticalVelocityUnits=m/s  SenseContactSignal=off  SensePenetrationDepth=off  SenseSeparationDistance=off  SenseNormalForceMagnitude=off  SenseFrictionalForceMagnitude=off  SenseNormalVelocity=off  SenseTangentialVelocity=off  SenseContactBaseRotation=off  SenseContactBaseTranslation=off  SenseContactFollowerRotation=off  SenseContactFollowerTranslation=off  ZeroCrossDetectContactStartAndEnd=off
  Spatial Contact Force1 : sm_lib/Forces and Torques/Spatial Contact Force  NormalForceType=SmoothSpringDamper  NormalStiffness=ctrl.commonModeContactStiffness/2  NormalStiffnessUnits=N/m  NormalDamping=ctrl.commonModeContactDamping/2  NormalDampingUnits=N/(m/s)  NormalTransitionRegionWidth=1e-3  NormalTransitionRegionWidthUnits=m  FrictionType=SmoothStickSlip  CoefficientOfStaticFriction=0.5  CoefficientOfDynamicFriction=0.3  FrictionalCriticalVelocity=0.02  FrictionalCriticalVelocityUnits=m/s  SenseContactSignal=off  SensePenetrationDepth=off  SenseSeparationDistance=off  SenseNormalForceMagnitude=off  SenseFrictionalForceMagnitude=off  SenseNormalVelocity=off  SenseTangentialVelocity=off  SenseContactBaseRotation=off  SenseContactBaseTranslation=off  SenseContactFollowerRotation=off  SenseContactFollowerTranslation=off  ZeroCrossDetectContactStartAndEnd=off
  Symmetry Diagnostics : Mux  Inputs=12
  Symmetry Diagnostics Terminator : Terminator
  World Frame1 : sm_lib/Frames and Transforms/World Frame
  Zero-Order Hold : ZeroOrderHold  SampleTime=base.Ts
  Connection Port : PMIOPort  Side=Left
  wires:
  PS-Simulink Converter/1 -> Fcn/1
  Mux/1 -> Zero-Order Hold/1
  Clock/1 -> Mux/1
  Zero-Order Hold/1 -> Common Wheel State Input/1, Coupled QP Input/1
  PS-Simulink Converter12/1 -> Fcn1/1
  Fcn1/1 -> Symmetry Diagnostics/1, Common Wheel State Input/2, Coupled QP Input/2, Scope/1
  Fcn/1 -> Symmetry Diagnostics/7, Coupled QP Input/8, Common Wheel State Input/8, Scope1/1
  PS-Simulink Converter13/1 -> Symmetry Diagnostics/2, Coupled QP Input/3, Common Wheel State Input/3
  PS-Simulink Converter16/1 -> Symmetry Diagnostics/3, Common Wheel State Input/4, Coupled QP Input/4
  PS-Simulink Converter17/1 -> Symmetry Diagnostics/4, Common Wheel State Input/5, Coupled QP Input/5
  PS-Simulink Converter14/1 -> Symmetry Diagnostics/5, Coupled QP Input/6, Common Wheel State Input/6
  PS-Simulink Converter15/1 -> Symmetry Diagnostics/6, Common Wheel State Input/7, Coupled QP Input/7
  PS-Simulink Converter1/1 -> Symmetry Diagnostics/8, Coupled QP Input/9, Common Wheel State Input/9
  PS-Simulink Converter2/1 -> Symmetry Diagnostics/9, Common Wheel State Input/10, Coupled QP Input/10
  PS-Simulink Converter9/1 -> Symmetry Diagnostics/10, Coupled QP Input/11, Common Wheel State Input/11
  PS-Simulink Converter10/1 -> Symmetry Diagnostics/11, Coupled QP Input/12, Common Wheel State Input/12
  PS-Simulink Converter11/1 -> Symmetry Diagnostics/12, Coupled QP Input/13, Common Wheel State Input/13
  Common Wheel State/1 -> Common Wheel Position LQR/1, NMPC State Split/1  "commonWheelStateSignal"
  Common Wheel Position LQR/1 -> Coupled QP Input/15, NMPC Reference Input/2  "wheelPositionLqrReference"
  NMPC State Split/1 -> NMPC Reference Input/1, NMPC Command Mux/1
  NMPC Solver/1 -> NMPC Previous Input/1, NMPC Command Mux/2  "nmpcBodyWrench"
  NMPC State Split/2 -> NMPC Solver/1, NMPC Solver/2  "baseWheelState"
  PS-Simulink Converter4/1 -> Mux/2  "x"
  PS-Simulink Converter6/1 -> Mux/3  "dy"
  PS-Simulink Converter18/1 -> Base Pitch from Quaternion/1  "baseQuaternion"
  Base Pitch from Quaternion/1 -> Mux/4
  PS-Simulink Converter3/1 -> Mux/5  "dx"
  PS-Simulink Converter7/1 -> Mux/6  "theta"
  PS-Simulink Converter19/1 -> Base Angular Velocity Split/1  "baseAngularVelocity"
  Base Angular Velocity Split/3 -> Mux/7
  Base Angular Velocity Split/1 -> Base Roll Rate Terminator/1
  Base Angular Velocity Split/2 -> Base Yaw Rate Terminator/1
  PS-Simulink Converter8/1 -> Base Lateral State/1  "dtheta"
  PS-Simulink Converter5/1 -> Base Lateral State/2  "y"
  Base Lateral State/1 -> Base Lateral State Terminator/1  "baseLateralState"
  Symmetry Diagnostics/1 -> Symmetry Diagnostics Terminator/1  "symmetryLegState"
  Common Wheel State Input/1 -> Common Wheel State/1
  Coupled QP Input/1 -> Coupled QP Input ZOH/1
  Coupled QP Input ZOH/1 -> Coupled QP/1
  Coupled QP/1 -> Coupled QP Split/1  "coupledQpSignal"
  Coupled QP Split/1 -> Left Torque Split/1
  Coupled QP Split/2 -> Right Torque Split/1
  Coupled QP Split/3 -> Coupled Slack Terminator/1
  Coupled QP Split/4 -> Coupled Feasible Terminator/1
  Coupled QP Split/5 -> Coupled Slack Norm Terminator/1
  Coupled QP Split/6 -> Coupled QP Status Terminator/1
  Coupled QP Split/7 -> Coupled Left Contact Force Terminator/1
  Coupled QP Split/8 -> Coupled Right Contact Force Terminator/1
  Coupled QP Split/9 -> Coupled Exit Flag Terminator/1
  Coupled QP Split/10 -> Coupled Dynamics Residual Terminator/1
  Coupled QP Split/11 -> Coupled Differential Qdd Terminator/1
  Coupled QP Split/12 -> Coupled Differential Qdd Command Terminator/1
  Coupled QP Split/13 -> Coupled Differential Torque Terminator/1
  Coupled QP Split/14 -> Coupled Differential Contact Force Terminator/1
  Coupled QP Split/15 -> Coupled Friction Margin Terminator/1
  Coupled QP Split/16 -> Coupled Torque Margin Terminator/1
  Coupled QP Split/17 -> Coupled Differential Wheel Position Terminator/1
  Coupled QP Split/18 -> Coupled Differential Wheel Velocity Terminator/1
  Coupled QP Split/19 -> Coupled Differential Wheel Acceleration Terminator/1
  Coupled QP Split/20 -> Coupled Differential Wheel Command Terminator/1
  Left Torque Split/1 -> Simulink-PS Converter5/1
  Right Torque Split/1 -> Simulink-PS Converter/1
  Left Torque Split/2 -> Simulink-PS Converter6/1
  Right Torque Split/2 -> Simulink-PS Converter1/1
  Left Torque Split/3 -> Simulink-PS Converter7/1
  Right Torque Split/3 -> Simulink-PS Converter4/1
  NMPC Previous Input/1 -> NMPC Reference Input/3
  NMPC Reference Input/1 -> NMPC Reference/1
  NMPC Reference/1 -> NMPC Reference Split/1
  NMPC Reference Split/1 -> NMPC Solver/3
  NMPC Reference Split/2 -> NMPC Solver/4
  NMPC Reference Split/3 -> NMPC Solver/5
  NMPC Solver/2 -> NMPC Command Mux/3  "nmpcStatus"
  NMPC Solver/3 -> NMPC Command Mux/4  "nmpcCpuTime"
  NMPC Command Mux/1 -> NMPC Command Guard/1
  NMPC Command Guard/1 -> NMPC Guard Split/1
  NMPC Guard Split/1 -> Coupled QP Input/14  "totalUpperCommand"
  NMPC Guard Split/2 -> NMPC Fault Terminator/1  "nmpcFault"
  connections:
  Brick Solid/RConn1 -- Rigid Transform10/LConn1 -- Rigid Transform5/LConn1 -- 6-DOF Joint/RConn1
  Brick Solid1/RConn1 -- Rigid Transform1/LConn1 -- Rigid Transform3/RConn1
  Rigid Transform3/LConn1 -- Right Revolute Joint/RConn1
  Right Revolute Joint/RConn2 -- PS-Simulink Converter/LConn1
  Rigid Transform2/LConn1 -- Revolute Joint1/RConn1
  Brick Solid2/RConn1 -- Rigid Transform4/LConn1 -- Rigid Transform2/RConn1
  PS-Simulink Converter1/LConn1 -- Revolute Joint1/RConn2
  Simulink-PS Converter/RConn1 -- Right Revolute Joint/LConn2
  Revolute Joint1/LConn1 -- Rigid Transform1/RConn1
  Simulink-PS Converter1/RConn1 -- Revolute Joint1/LConn2
  Cylindrical Solid/RConn1 -- Revolute Joint2/RConn1
  World Frame1/RConn1 -- Solver Configuration/RConn1 -- Rigid Transform/LConn1 -- Brick Solid3/RConn1 -- Mechanism Configuration/RConn1
  6-DOF Joint/LConn1 -- Rigid Transform/RConn1
  Revolute Joint2/LConn1 -- Rigid Transform4/RConn1
  Spatial Contact Force/RConn1 -- Spatial Contact Force1/RConn1 -- Brick Solid3/LConn1
  Simulink-PS Converter4/RConn1 -- Revolute Joint2/LConn2
  PS-Simulink Converter2/LConn1 -- Revolute Joint2/RConn2
  6-DOF Joint/RConn2 -- PS-Simulink Converter4/LConn1
  Rigid Transform5/RConn1 -- Right Revolute Joint/LConn1
  PS-Simulink Converter9/LConn1 -- Right Revolute Joint/RConn3
  Revolute Joint1/RConn3 -- PS-Simulink Converter10/LConn1
  PS-Simulink Converter11/LConn1 -- Revolute Joint2/RConn3
  Rigid Transform9/LConn1 -- Brick Solid5/RConn1 -- Rigid Transform7/RConn1
  Rigid Transform6/LConn1 -- Rigid Transform8/RConn1 -- Brick Solid4/RConn1
  Simulink-PS Converter6/RConn1 -- Revolute Joint4/LConn2
  Revolute Joint5/LConn1 -- Rigid Transform9/RConn1
  Simulink-PS Converter7/RConn1 -- Revolute Joint5/LConn2
  Left Revolute Joint3/RConn2 -- PS-Simulink Converter12/LConn1
  Rigid Transform8/LConn1 -- Left Revolute Joint3/RConn1
  PS-Simulink Converter13/LConn1 -- Revolute Joint4/RConn2
  PS-Simulink Converter16/LConn1 -- Revolute Joint5/RConn2
  Revolute Joint4/RConn3 -- PS-Simulink Converter14/LConn1
  Cylindrical Solid1/RConn1 -- Revolute Joint5/RConn1
  PS-Simulink Converter17/LConn1 -- Left Revolute Joint3/RConn3
  Rigid Transform10/RConn1 -- Left Revolute Joint3/LConn1
  Simulink-PS Converter5/RConn1 -- Left Revolute Joint3/LConn2
  Revolute Joint4/LConn1 -- Rigid Transform6/RConn1
  PS-Simulink Converter15/LConn1 -- Revolute Joint5/RConn3
  Rigid Transform7/LConn1 -- Revolute Joint4/RConn1
  Cylindrical Solid/LConn1 -- Spatial Contact Force/LConn1
  Cylindrical Solid1/LConn1 -- Spatial Contact Force1/LConn1
  PS-Simulink Converter5/LConn1 -- 6-DOF Joint/RConn7
  6-DOF Joint/RConn3 -- PS-Simulink Converter3/LConn1
  6-DOF Joint/RConn4 -- PS-Simulink Converter6/LConn1
  6-DOF Joint/RConn6 -- PS-Simulink Converter8/LConn1
  PS-Simulink Converter7/LConn1 -- 6-DOF Joint/RConn5
  6-DOF Joint/RConn8 -- PS-Simulink Converter18/LConn1
  6-DOF Joint/RConn9 -- PS-Simulink Converter19/LConn1
  Simulink-PS Converter8/RConn1 -- 6-DOF Joint/LConn2
